simulink subsystem "PieroControladoS"  (R2023b)
settings: Solver=VariableStepAuto  StartTime=0.0  StopTime=10.0  RelTol=1e-3
settings Model: Creator=adria  LastModifiedBy=adria

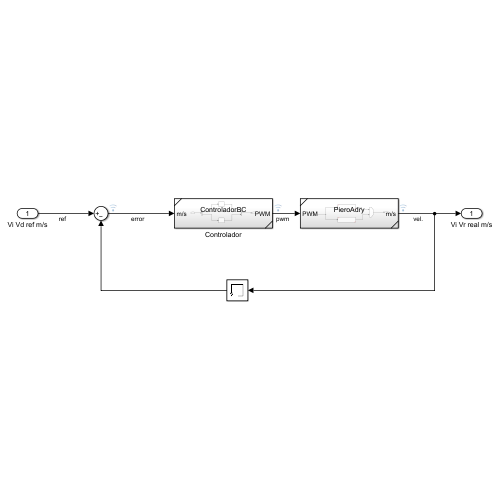
[thumbnail: Simulink's stored preview of the top-level diagram]
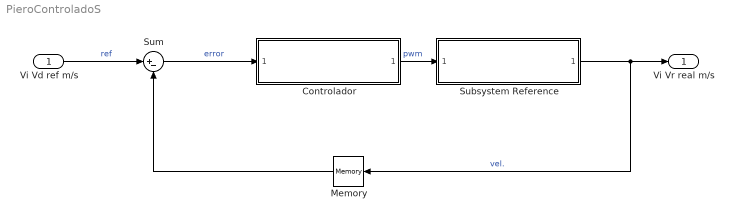
== system PieroControladoS ==
  Vi Vd ref m/s : Inport  OutDataTypeStr=double  PortDimensions=2
  Controlador : Subsystem  ReferencedSubsystem=ControladorBC
  Memory : Memory
  Subsystem Reference : Subsystem  ReferencedSubsystem=PieroAdry
  Sum : Sum  Inputs=|+-
  Vi Vr real m/s : Outport  OutDataTypeStr=double  PortDimensions=2
  wires:
  Sum/1 -> Controlador/1  "error"
  Subsystem Reference/1 -> Vi Vr real m/s/1, Memory/1  "vel."
  Controlador/1 -> Subsystem Reference/1  "pwm"
  Vi Vd ref m/s/1 -> Sum/1  "ref"
  Memory/1 -> Sum/2
